simulink model "Systemmodel"  (R2018b)
settings: Solver=VariableStepAuto  StartTime=0.0  StopTime=Endtime  RelTol=1e-3
values from neighbouring files (symbols this model uses):
  alpha_A = (2^n - 1)/(V_A_max - V_A_min)    (= 204.6)    [Systemmodel_sim.m]
  alpha_i = 5/37.5    (= 0.133333333333)    [Systemmodel_sim.m]
  alpha_P = 100/(2^m - 1)    (= 0.392156862745)    [Systemmodel_sim.m]
  alpha_T = 1.5/1000    (= 0.0015)    [Systemmodel_sim.m]
  D = 6.0e-5    (= 6e-05)    [Systemmodel_sim.m]
  Ji = 1.3e-3    (= 0.0013)    [Systemmodel_sim.m]
  Jm = 0.11e-3    (= 0.00011)    [Systemmodel_sim.m]
  Ke = 7.16e-2    (= 0.0716)    [Systemmodel_sim.m]
  Kt = 7.2e-2    (= 0.072)    [Systemmodel_sim.m]
  L = 0.2    [Systemmodel_sim.m]
  m = 8    [Systemmodel_sim.m]
  R = 5.7    [Systemmodel_sim.m]
  smp = 0.001    [Systemmodel_sim.m]
  u_max = 100    [Systemmodel_sim.m]
  u_min = 0    [Systemmodel_sim.m]
  V_A_max = 5    [Systemmodel_sim.m]
  V_A_min = 0    [Systemmodel_sim.m]
  Vin = 24    [Systemmodel_sim.m]
settings Model: Creator=nharada  LastModifiedBy=nharada

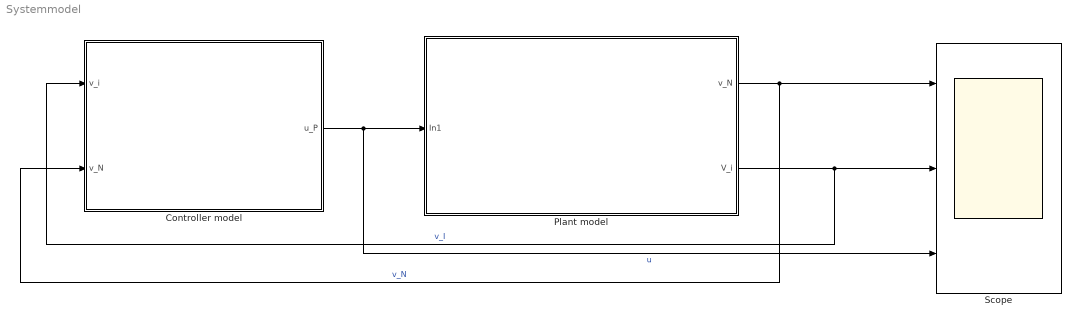
== system Systemmodel ==
  Controller model : Subsystem
  "Plant model " : Subsystem
  Scope : Scope  NumInputPorts=3
  wires:
  "Plant model "/1("v_N ") -> Controller model/2(v_N), Scope/1  "v_N"
  Controller model/1(u_P) -> Scope/3, "Plant model "/1(In1)  "u"
  "Plant model "/2(V_i) -> Controller model/1(v_i), Scope/2  "v_I"

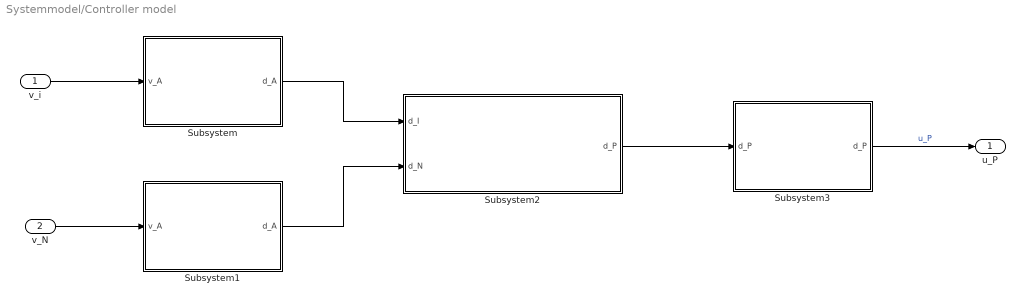
== system Systemmodel/Controller model ==
  v_i : Inport
  v_N : Inport  Port=2
  Subsystem : Subsystem
  Subsystem1 : Subsystem
  Subsystem2 : Subsystem
  Subsystem3 : Subsystem
  u_P : Outport
  wires:
  Subsystem3/1(d_P) -> u_P/1  "u_P"
  Subsystem2/1(d_P) -> Subsystem3/1("d_P ")
  v_N/1 -> Subsystem1/1(v_A)
  Subsystem/1(d_A) -> Subsystem2/1(d_I)
  Subsystem1/1(d_A) -> Subsystem2/2(d_N)
  v_i/1 -> Subsystem/1(v_A)

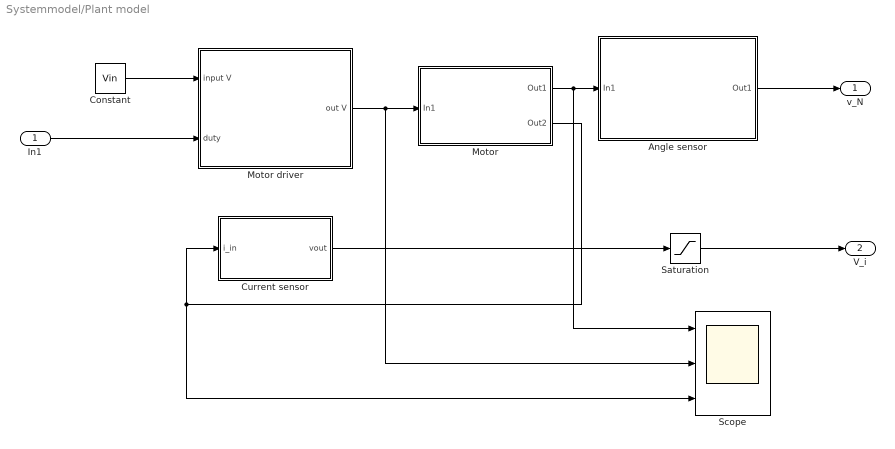
== system Systemmodel/Plant model  ==
  In1 : Inport
  Angle sensor : Subsystem
  Constant : Constant  Value=Vin
  Current sensor : Subsystem
  Motor : Subsystem
  Motor driver : Subsystem
  Saturation : Saturate  UpperLimit=5  LowerLimit=0
  Scope : Scope  NumInputPorts=3
  "v_N " : Outport
  V_i : Outport  Port=2
  wires:
  Current sensor/1(vout) -> Saturation/1
  Constant/1 -> Motor driver/1(input V)
  Motor driver/1(out V) -> Scope/2, Motor/1(In1)
  Motor/2(Out2) -> Current sensor/1(i_in), Scope/3
  Motor/1(Out1) -> Scope/1, Angle sensor/1(In1)
  In1/1 -> Motor driver/2(duty)
  Angle sensor/1(Out1) -> "v_N "/1
  Saturation/1 -> V_i/1

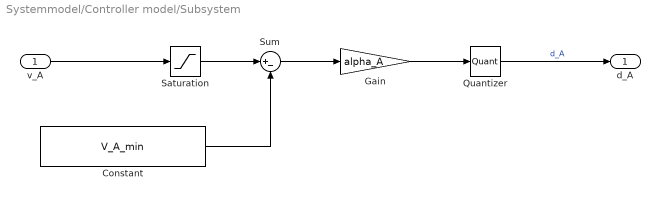
== system Systemmodel/Controller model/Subsystem ==
  v_A : Inport
  Constant : Constant  Value=V_A_min  SampleTime=smp
  Gain : Gain  Gain=alpha_A
  Quantizer : Quantizer  QuantizationInterval=1
  Saturation : Saturate  UpperLimit=V_A_max  LowerLimit=V_A_min
  Sum : Sum  Inputs=|+-
  d_A : Outport
  wires:
  Saturation/1 -> Sum/1
  Sum/1 -> Gain/1
  Gain/1 -> Quantizer/1
  v_A/1 -> Saturation/1
  Quantizer/1 -> d_A/1  "d_A"
  Constant/1 -> Sum/2

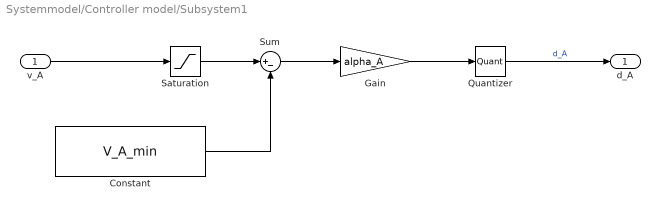
== system Systemmodel/Controller model/Subsystem1 ==
  v_A : Inport
  Constant : Constant  Value=V_A_min  SampleTime=smp
  Gain : Gain  Gain=alpha_A
  Quantizer : Quantizer  QuantizationInterval=1
  Saturation : Saturate  UpperLimit=V_A_max  LowerLimit=V_A_min
  Sum : Sum  Inputs=|+-
  d_A : Outport
  wires:
  Saturation/1 -> Sum/1
  Sum/1 -> Gain/1
  Gain/1 -> Quantizer/1
  v_A/1 -> Saturation/1
  Quantizer/1 -> d_A/1  "d_A"
  Constant/1 -> Sum/2

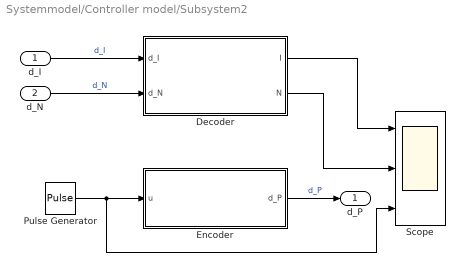
== system Systemmodel/Controller model/Subsystem2 ==
  d_I : Inport
  d_N : Inport  Port=2
  Decoder : Subsystem
  Encoder : Subsystem
  Pulse Generator : DiscretePulseGenerator  PulseType=Time based  Amplitude=100  Period=30  PulseWidth=50
  Scope : Scope  NumInputPorts=3
  d_P : Outport
  wires:
  Pulse Generator/1 -> Scope/3, Encoder/1(u)
  Decoder/2(N) -> Scope/2
  d_N/1 -> Decoder/2(d_N)  "d_N"
  Decoder/1(I) -> Scope/1
  d_I/1 -> Decoder/1(d_I)  "d_I"
  Encoder/1(d_P) -> d_P/1  "d_P"

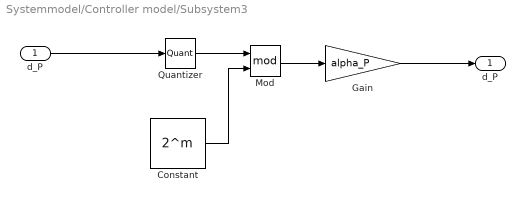
== system Systemmodel/Controller model/Subsystem3 ==
  "d_P " : Inport
  Constant : Constant  Value=2^m  SampleTime=smp
  Gain : Gain  Gain=alpha_P
  Mod : Math  Operator=mod  SaturateOnIntegerOverflow=on
  Quantizer : Quantizer  QuantizationInterval=1
  d_P : Outport
  wires:
  Quantizer/1 -> Mod/1
  Constant/1 -> Mod/2
  Mod/1 -> Gain/1
  Gain/1 -> d_P/1
  "d_P "/1 -> Quantizer/1

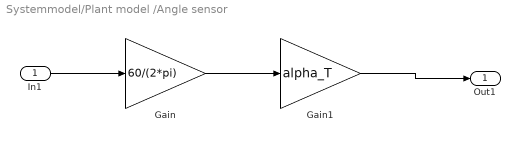
== system Systemmodel/Plant model /Angle sensor ==
  In1 : Inport
  Gain : Gain  Gain=60/(2*pi)
  Gain1 : Gain  Gain=alpha_T
  Out1 : Outport
  wires:
  In1/1 -> Gain/1
  Gain/1 -> Gain1/1
  Gain1/1 -> Out1/1

== system Systemmodel/Plant model /Current sensor ==
  i_in : Inport
  Gain : Gain  Gain=alpha_i
  vout : Outport
  wires:
  Gain/1 -> vout/1  "vout"
  i_in/1 -> Gain/1

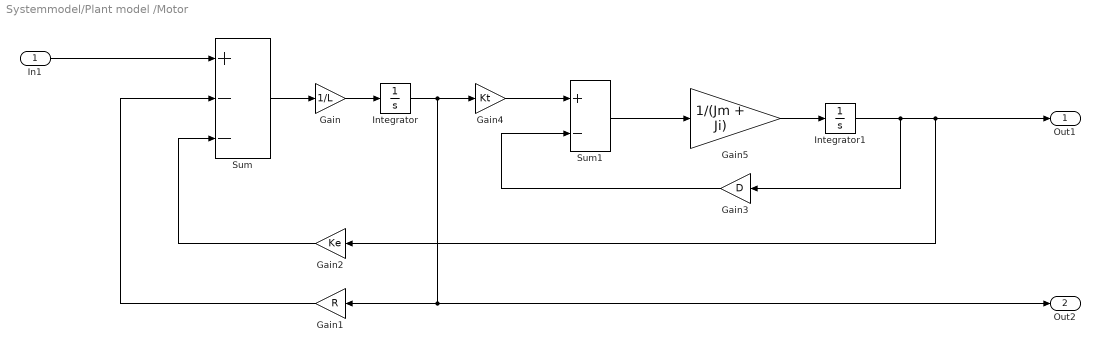
== system Systemmodel/Plant model /Motor ==
  In1 : Inport
  Gain : Gain  Gain=1/L
  Gain1 : Gain  Gain=R
  Gain2 : Gain  Gain=Ke
  Gain3 : Gain  Gain=D
  Gain4 : Gain  Gain=Kt
  Gain5 : Gain  Gain=1/(Jm + Ji)
  Integrator : Integrator
  Integrator1 : Integrator
  Sum : Sum  Inputs=+--
  Sum1 : Sum  Inputs=+-
  Out1 : Outport
  Out2 : Outport  Port=2
  wires:
  Gain1/1 -> Sum/2
  Sum/1 -> Gain/1
  Gain3/1 -> Sum1/2
  Gain2/1 -> Sum/3
  Gain/1 -> Integrator/1
  Integrator1/1 -> Gain3/1, Out1/1, Gain2/1
  Integrator/1 -> Gain4/1, Out2/1, Gain1/1
  Sum1/1 -> Gain5/1
  Gain5/1 -> Integrator1/1
  Gain4/1 -> Sum1/1
  In1/1 -> Sum/1

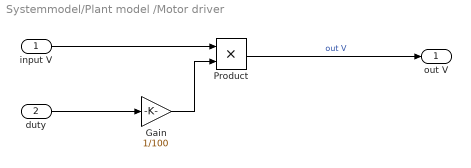
== system Systemmodel/Plant model /Motor driver ==
  input V : Inport
  duty : Inport  Port=2
  Gain : Gain  Gain=1/100
  Product : Product
  out V : Outport
  wires:
  Gain/1 -> Product/2
  input V/1 -> Product/1
  Product/1 -> out V/1  "out V"
  duty/1 -> Gain/1

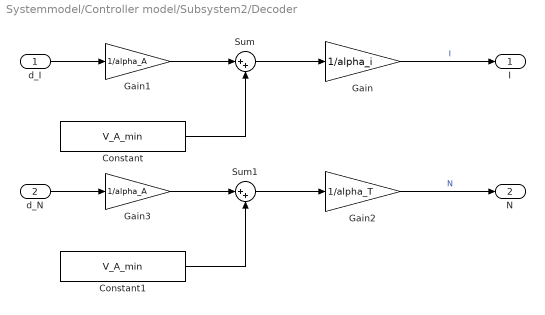
== system Systemmodel/Controller model/Subsystem2/Decoder ==
  d_I : Inport
  d_N : Inport  Port=2
  Constant : Constant  Value=V_A_min  SampleTime=smp
  Constant1 : Constant  Value=V_A_min  SampleTime=smp
  Gain : Gain  Gain=1/alpha_i
  Gain1 : Gain  Gain=1/alpha_A
  Gain2 : Gain  Gain=1/alpha_T
  Gain3 : Gain  Gain=1/alpha_A
  Sum : Sum  Inputs=|++
  Sum1 : Sum  Inputs=|++
  I : Outport
  N : Outport  Port=2
  wires:
  Gain2/1 -> N/1  "N"
  Gain/1 -> I/1  "I"
  Gain1/1 -> Sum/1
  d_N/1 -> Gain3/1
  Gain3/1 -> Sum1/1
  d_I/1 -> Gain1/1
  Sum/1 -> Gain/1
  Sum1/1 -> Gain2/1
  Constant1/1 -> Sum1/2
  Constant/1 -> Sum/2

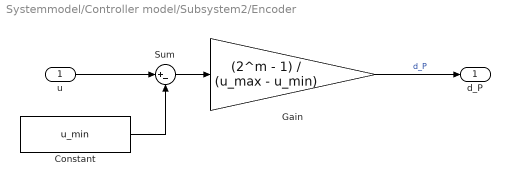
== system Systemmodel/Controller model/Subsystem2/Encoder ==
  u : Inport
  Constant : Constant  Value=u_min  SampleTime=smp
  Gain : Gain  Gain=(2^m - 1) / (u_max - u_min)
  Sum : Sum  Inputs=|+-
  d_P : Outport
  wires:
  Sum/1 -> Gain/1
  u/1 -> Sum/1
  Gain/1 -> d_P/1  "d_P"
  Constant/1 -> Sum/2
